simulink model "single_track_func"  (R2022b)
settings: Solver=VariableStepAuto  StartTime=0.0  StopTime=10.0  RelTol=1e-3
settings Model: Creator=ashkan  LastModifiedBy=ashkan

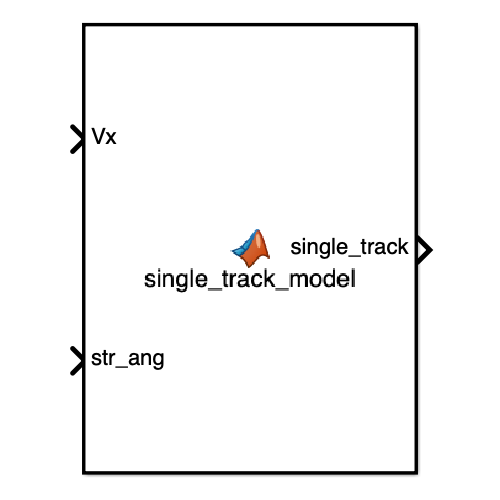
[thumbnail: Simulink's stored preview of the top-level diagram]
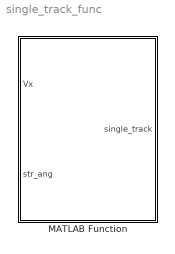
== system single_track_func ==
  MATLAB Function : MATLAB Function  TreatAsAtomicUnit=on

== matlab function single_track_func/MATLAB Function ==
  data: single_track output; Vx input; str_ang input; vehicle_data parameter
function single_track = single_track_model(Vx , str_ang , vehicle_data)

    

   % here is some simplified parameters :)
   m = vehicle_data.vehicle.m;
   a = vehicle_data.vehicle.Lf;
   b = vehicle_data.vehicle.Lr;
   izz = vehicle_data.vehicle.i_zz;
   g = vehicle_data.vehicle.g;
   L = vehicle_data.vehicle.L;
   mu = 0.2;  % --> should come from scenario
   Caf = vehicle_data.front_suspension.Ks_f ;
   Car = vehicle_data.rear_suspension.Ks_r;


   beta_ss  = (((2*b*L*Caf*Car)- (m*a*Cf*Vx^2))/((2*Caf*Car*L^2)-(m*(a*Caf - b*Car)*Vx^2)))*str_ang;
   beta_lim = atan(0.02*mu*g);
   beta_d = min(beta_ss , beta_lim);

   rss   = ((2*L*Caf*Car*Vx)/((2*Caf*Car*L^2)-(m*(a*Caf - b*Car)*Vx^2)))*str_ang;
   r_lim = 0.85*abs(mu*g / Vx);
   r_d = min(rss , r_lim);
   
   single_track = ;


end
